simulink model "Three_phase_inverter"  (R2021a)
settings: Solver=VariableStepAuto  StartTime=0.0  StopTime=.1  RelTol=1e-3
libraries: spsIGBTDiodeLib x6, spsVoltageMeasurementLib x6, spsCurrentMeasurementLib x3, spsSeriesRLCBranchLib x3, spsDCVoltageSourceLib x1, spsTriangleGeneratorLib x1, spspowerguiLib x1
settings Model: Creator=Himel Khan  LastModifiedBy=User

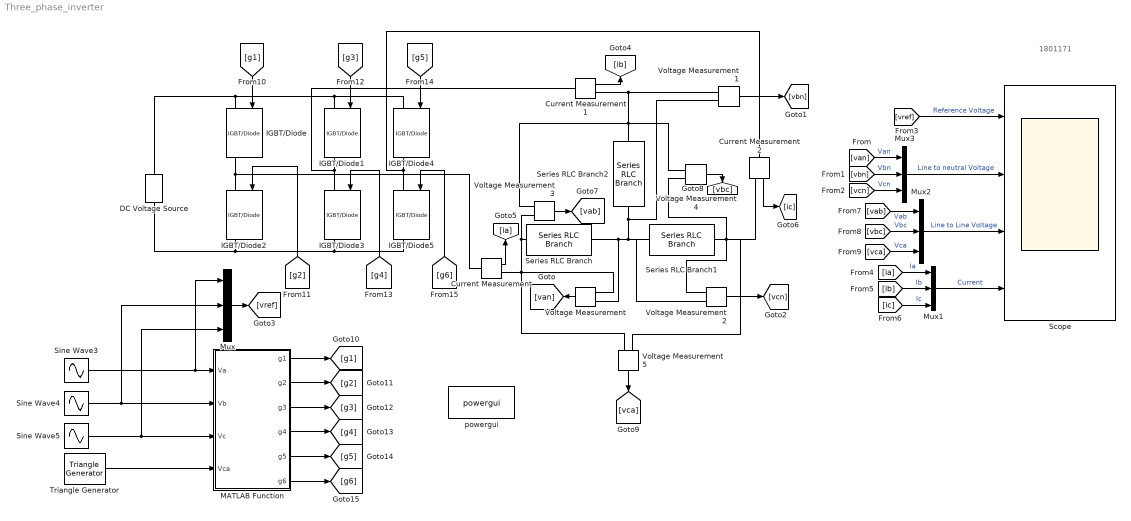
== system Three_phase_inverter ==
  note: 1801171
  Current Measurement : spsCurrentMeasurementLib/Current Measurement  PhasorSimulation=off  OutputType=Complex  PSBequivalent=0
  Current Measurement1 : spsCurrentMeasurementLib/Current Measurement  PhasorSimulation=off  OutputType=Complex  PSBequivalent=0
  Current Measurement2 : spsCurrentMeasurementLib/Current Measurement  PhasorSimulation=off  OutputType=Complex  PSBequivalent=0
  DC Voltage Source : spsDCVoltageSourceLib/DC Voltage Source  Amplitude=50  Measurements=None
  IGBT/Diode{,1..5} (6 alike) : spsIGBTDiodeLib/IGBT//Diode  Ron=1e-3  Rs=1e5  Cs=inf  Measurements=on
  MATLAB Function : MATLAB Function  TreatAsAtomicUnit=on
  Mux{,1..3} (4 alike) : Mux  Inputs=3
  Scope : Scope  NumInputPorts=4
  Series RLC Branch : spsSeriesRLCBranchLib/Series RLC Branch  LConnTagsString=__new0  RConnTagsString=__new0  BranchType=RL  Resistance=5  Inductance=100e-3  SetiL0=off  InitialCurrent=0  Capacitance=1e-6  Setx0=off  InitialVoltage=0  Measurements=None
  Series RLC Branch1 : spsSeriesRLCBranchLib/Series RLC Branch  LConnTagsString=__new0  RConnTagsString=__new0  BranchType=RL  Resistance=5  Inductance=100e-3  SetiL0=off  InitialCurrent=0  Capacitance=1e-6  Setx0=off  InitialVoltage=0  Measurements=None
  Series RLC Branch2 : spsSeriesRLCBranchLib/Series RLC Branch  LConnTagsString=__new0  RConnTagsString=__new0  BranchType=RL  Resistance=5  Inductance=100e-3  SetiL0=off  InitialCurrent=0  Capacitance=1e-6  Setx0=off  InitialVoltage=0  Measurements=None
  Sine Wave3 : Sin  Frequency=2*pi*50  SampleTime=0
  Sine Wave4 : Sin  Frequency=2*pi*50  Phase=-2*pi/3  SampleTime=0
  Sine Wave5 : Sin  Frequency=2*pi*50  Phase=-4*pi/3  SampleTime=0
  Triangle Generator : spsTriangleGeneratorLib/Triangle Generator  Freq=1e3  Phase=0  Ts=0
  Voltage Measurement{,1..5} (6 alike) : spsVoltageMeasurementLib/Voltage Measurement  PhasorSimulation=off  OutputType=Complex  PSBequivalent=0
  powergui : spspowerguiLib/powergui  Priority=1  SimulationMode=Discrete  SampleTime=50e-6  frequency=60  Iterations=50  frequencyindice=0  Pbase=100e6  ErrMax=1e-4  UnitsV=kV  UnitsW=MW  buscounter=0  FunctionMessages=off  echomessages=off  EnableUseOfTLC=off  CurrentSourceSwitches=off  DisableSnubberDevices=off  DisableRonSwitches=off  DisableVfSwitches=off  DisplayEquations=off  AutomaticDiscreteSolvers=off  SolverType=Tustin/Backward Euler (TBE)  Interpol=off  ExternalGateDelay=off  methode=off  Ts=100  x0status=blocks  SPID=on  SwTol=0  HookPort=off  NonlinearTolerance=1e-4  nMaxIteration=100  ContinueOnMaxIteration=off  RestoreLinks=warning  ResistiveCurrentMeasurement=off  Frange=[0:2:500]  Ylog=off  Xlog=on  ShowGrid=off  save=off  variable=ZData  structure=0  ZoomFFT=off  StartTime=0.0  cycles=1  DisplayStyle=1  fundamental=60  FreqAxis=off  MaxFrequency=1000  frequencyindicesteady=1  RmsSteady=1  display=off
  wires:
  Sine Wave4/1 -> MATLAB Function/2(Vb), Mux/2
  Sine Wave5/1 -> Mux/3, MATLAB Function/3(Vc)
  Voltage Measurement/1 -> [van]
  Voltage Measurement1/1 -> [vbn]
  Voltage Measurement2/1 -> [vcn]
  Sine Wave3/1 -> Mux/1, MATLAB Function/1(Va)
  Mux/1 -> [vref]
  [vref] -> Scope/1  "Reference Voltage"
  Triangle Generator/1 -> MATLAB Function/4(Vca)
  Mux1/1 -> Scope/4  "Current"
  [ib] -> Mux1/2  "Ib"
  [ia] -> Mux1/1  "Ia"
  [ic] -> Mux1/3  "Ic"
  Current Measurement1/1 -> [ib]
  Current Measurement/1 -> [ia]
  Current Measurement2/1 -> [ic]
  Voltage Measurement3/1 -> [vab]
  Voltage Measurement4/1 -> [vbc]
  Voltage Measurement5/1 -> [vca]
  MATLAB Function/1(g1) -> [g1]
  [g1] -> IGBT/Diode/1
  MATLAB Function/2(g2) -> [g2]
  [g2] -> IGBT/Diode2/1
  MATLAB Function/3(g3) -> [g3]
  [g3] -> IGBT/Diode1/1
  MATLAB Function/4(g4) -> [g4]
  [g4] -> IGBT/Diode3/1
  MATLAB Function/5(g5) -> [g5]
  [g5] -> IGBT/Diode4/1
  MATLAB Function/6(g6) -> [g6]
  [g6] -> IGBT/Diode5/1
  [vbc] -> Mux2/2  "Vbc"
  [vca] -> Mux2/3  "Vca"
  [vab] -> Mux2/1  "Vab"
  Mux2/1 -> Scope/3  "Line to Line Voltage"
  [van] -> Mux3/1  "Van"
  [vbn] -> Mux3/2  "Vbn"
  [vcn] -> Mux3/3  "Vcn"
  Mux3/1 -> Scope/2  "Line to neutral Voltage"
  connections:
  IGBT/Diode2/LConn1 -- IGBT/Diode/RConn1 -- Current Measurement/LConn1
  IGBT/Diode/LConn1 -- IGBT/Diode4/LConn1 -- IGBT/Diode1/LConn1 -- DC Voltage Source/RConn1
  IGBT/Diode3/LConn1 -- Current Measurement1/LConn1 -- IGBT/Diode1/RConn1
  Series RLC Branch1/LConn1 -- Voltage Measurement5/LConn1 -- Current Measurement2/RConn1 -- Voltage Measurement4/LConn2 -- Voltage Measurement2/LConn1
  IGBT/Diode5/RConn1 -- IGBT/Diode3/RConn1 -- DC Voltage Source/LConn1 -- IGBT/Diode2/RConn1
  Series RLC Branch/RConn1 -- Voltage Measurement/LConn2 -- Voltage Measurement2/LConn2 -- Series RLC Branch1/RConn1 -- Voltage Measurement1/LConn2 -- Series RLC Branch2/RConn1
  Voltage Measurement/LConn1 -- Series RLC Branch/LConn1 -- Voltage Measurement3/LConn1 -- Voltage Measurement5/LConn2 -- Current Measurement/RConn1
  Voltage Measurement1/LConn1 -- Voltage Measurement4/LConn1 -- Voltage Measurement3/LConn2 -- Series RLC Branch2/LConn1 -- Current Measurement1/RConn1
  IGBT/Diode5/LConn1 -- Current Measurement2/LConn1 -- IGBT/Diode4/RConn1

== matlab function Three_phase_inverter/MATLAB Function ==
  data: Va input; g1 output; Vb input; Vc input; g2 output; g3 output; g4 output; g5 output; g6 output; Vca input
function [g1,g2,g3,g4, g5,g6] = fcn(Va, Vb, Vc,Vca)

if Va>=Vca
    g1=1;
    g2=0;
else
    g1=0;
    g2=1;
end
if Vb>=Vca
    g3=1;
    g4=0;
else
    g3=0;
    g4=1;
end
if Vc>=Vca
    g5=1;
    g6=0;
else
    g5=0;
    g6=1;
end
end
